simulink model "DPP_open_loop"  (R2019b)
settings: Solver=VariableStepAuto  StartTime=0.0  StopTime=3  RelTol=1e-5  EnableMultiTasking=on
libraries: powerlib x19, re_lib x2, eePwmGenerator x2, simulink x1
settings Model: Creator=Rodney Tan  LastModifiedBy=lward
settings SolverCC: ConcurrentTasks=on  ZeroCrossControl=DisableAll  AlgebraicLoopSolver=LineSearch
settings DataIOCC: LimitDataPoints=on  SaveFormat=Array  ReturnWorkspaceOutputs=off
settings OptimizationCC: LifeSpan=inf
settings DebuggingCC: SFUnexpectedBacktrackingDiag=warning  SFNoUnconditionalDefaultTransitionDiag=warning  ArithmeticOperatorsInVariantConditions=warning
settings HardwareCC: ProdBitPerPointer=32  ProdBitPerSizeT=32  ProdBitPerPtrDiffT=32  ProdLargestAtomicFloat=None  ProdIntDivRoundTo=Undefined  ProdEndianess=Unspecified  ProdWordSize=32  ProdHWDeviceType=32-bit Generic
settings ModelReferenceCC: PropagateSignalLabelsOutOfModel=off
settings SFSimCC: SimUseLocalCustomCode=off  CustomCodeUndefinedFunction=UseInterfaceOnly
settings RTWCC: RTWUseLocalCustomCode=off
settings CodeAppCC: StateflowObjectComments=on
settings GRTTargetCC: TargetLangStandard=C89/C90 (ANSI)  GeneratePreprocessorConditionals=Disable all
settings ConfigComp: CovMetricSettings=dw  CovHtmlReporting=on  CovSaveCumulativeToWorkspaceVar=on  CovSaveSingleToWorkspaceVar=on  CovExternalEMLEnable=off
settings SimscapeCC: SimscapeNormalizeSystem=off

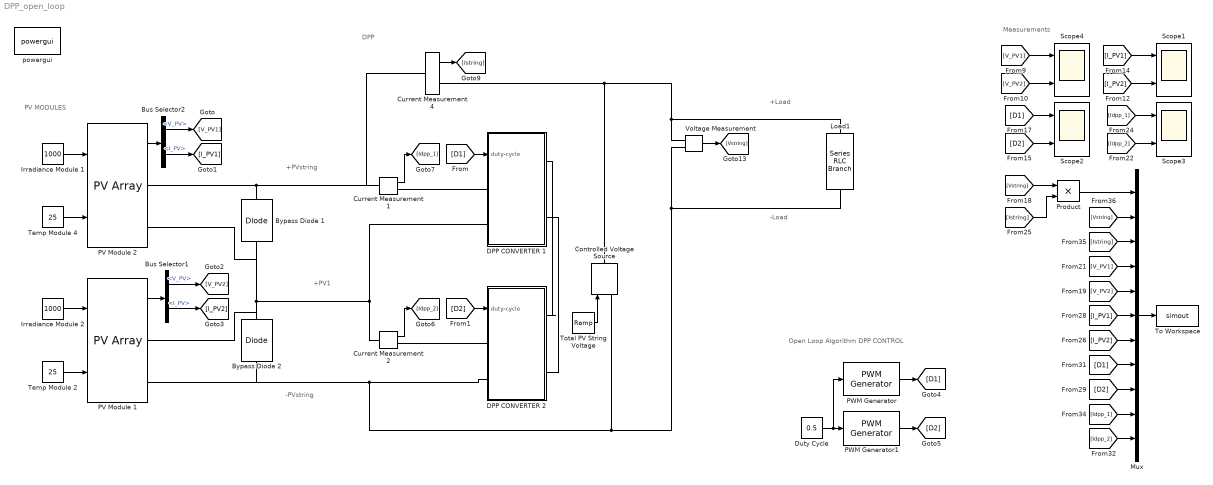
== system DPP_open_loop ==
  note: PV MODULES
  note: DPP
  note: +PV1
  note: +PVstring
  note: +Load
  note: -Load
  note: Measurements
  note: -PVstring
  note: Open Loop Algorithm
      | DPP CONTROL
  Bus Selector1 : BusSelector  OutputSignals=V_PV,I_PV
  Bus Selector2 : BusSelector  OutputSignals=V_PV,I_PV
  Bypass Diode 1 : powerlib/Power Electronics/Diode  Ron=0  Lon=0  Vf=0.8  IC=0  UseSnubber=off  Rs=0  Cs=0  Measurements=off
      settings: SourceProductName=Simscape Electrical
  Bypass Diode 2 : powerlib/Power Electronics/Diode  Ron=0  Lon=0  Vf=0.8  IC=0  UseSnubber=off  Rs=0  Cs=0  Measurements=off
      settings: SourceProductName=Simscape Electrical
  Controlled Voltage Source : powerlib/Electrical Sources/Controlled Voltage Source  Initialize=on  Source_Type=DC  Amplitude=0  Phase=0  Frequency=0  Measurements=None
      settings: SourceProductName=Simscape Electrical
  Current Measurement1 : powerlib/Measurements/Current Measurement  PhasorSimulation=off  OutputType=Complex  PSBequivalent=0
      settings: SourceProductName=Simscape Electrical
  Current Measurement2 : powerlib/Measurements/Current Measurement  PhasorSimulation=off  OutputType=Complex  PSBequivalent=0
      settings: SourceProductName=Simscape Electrical
  Current Measurement4 : powerlib/Measurements/Current Measurement  PhasorSimulation=off  OutputType=Complex  PSBequivalent=0
      settings: SourceProductName=Simscape Electrical
  DPP CONVERTER 1 : Subsystem
  DPP CONVERTER 2 : Subsystem
  Duty Cycle : Constant  Value=0.5
  Irradiance Module 1 : Constant  Value=1000
  Irradiance Module 2 : Constant  Value=1000
  Load1 : powerlib/Elements/Series RLC Branch  LConnTagsString=__new0  RConnTagsString=__new0  BranchType=R  Resistance=40  Inductance=1e-3  SetiL0=off  InitialCurrent=0  Capacitance=100e-6  Setx0=off  InitialVoltage=0  Measurements=None
      settings: SourceProductName=Simscape Electrical
  Mux : Mux  Inputs=11
  PV Module 1 : re_lib/Solar/PV Array  Npar=1  Nser=1  PlotType=array @ 1000 W/m2 & specified temperatures  S_vec="[ 1000  500  100 ]"  Temp_C_vec="[ 45 25  ]"  ModuleName=Renogy RNG-175D  PlotWhenSelected=off  Pm=175.062  Ncell=72  Voc=44.2  Isc=5.25  Vm=35.8  Im=4.89  beta_Voc_pc=-0.386  alpha_Isc_pc=0.0436  beta_Voc=-0.17061  alpha_Isc=0.002289  IL=5.2606  I0=4.127e-10  nI=1.0278  Rsh=408.404  Rs=0.58188  BAL=off  Tc=1e-6  Tfilter=5e-5
      settings: SourceProductName=Simscape Electrical
  PV Module 2 : re_lib/Solar/PV Array  Npar=1  Nser=1  PlotType=array @ 1000 W/m2 & specified temperatures  S_vec="[ 1000  500  100 ]"  Temp_C_vec="[ 45 25  ]"  ModuleName=Renogy RNG-175D  PlotWhenSelected=off  Pm=175.062  Ncell=72  Voc=44.2  Isc=5.25  Vm=35.8  Im=4.89  beta_Voc_pc=-0.386  alpha_Isc_pc=0.0436  beta_Voc=-0.17061  alpha_Isc=0.002289  IL=5.2606  I0=4.127e-10  nI=1.0278  Rsh=408.404  Rs=0.58188  BAL=off  Tc=1e-6  Tfilter=5e-5
      settings: SourceProductName=Simscape Electrical
  PWM Generator : eePwmGenerator/PWM Generator  CarrCount=Up  Tper=0.0001  Ts=1e-5
      settings: SourceProductName=Simscape Electrical
  PWM Generator1 : eePwmGenerator/PWM Generator  CarrCount=Up  Tper=0.0001  Ts=1e-5
      settings: SourceProductName=Simscape Electrical
  Product : Product
  Scope{1..4} (4 alike) : Scope  NumInputPorts=2
  Temp Module 2 : Constant  Value=25
  Temp Module 4 : Constant  Value=25
  To Workspace : ToWorkspace  VariableName=simout  SampleTime=-1
  Total PV String Voltage : simulink/Sources/Ramp  slope=50  start=0  InitialOutput=0
  Voltage Measurement : powerlib/Measurements/Voltage Measurement  PhasorSimulation=off  OutputType=Complex  PSBequivalent=0
      settings: SourceProductName=Simscape Electrical
  powergui : powerlib/powergui  Priority=1  SimulationMode=Continuous  SampleTime=1e-6  frequency=60  Iterations=50  frequencyindice=0  Pbase=100e6  ErrMax=1e-4  UnitsV=kV  UnitsW=MW  buscounter=0  FunctionMessages=off  echomessages=off  EnableUseOfTLC=off  CurrentSourceSwitches=off  DisableSnubberDevices=off  DisableRonSwitches=off  DisableVfSwitches=off  DisplayEquations=off  AutomaticDiscreteSolvers=off  SolverType=Tustin/Backward Euler (TBE)  Interpol=off  ExternalGateDelay=off  methode=off  Ts=100  x0status=blocks  SPID=off  SwTol=0  HookPort=off  NonlinearTolerance=1e-4  nMaxIteration=100  ContinueOnMaxIteration=off  RestoreLinks=warning  ResistiveCurrentMeasurement=off  Frange=[0:2:500]  Ylog=off  Xlog=on  ShowGrid=off  save=off  variable=ZData  structure=0  ZoomFFT=off  StartTime=0.0  cycles=1  DisplayStyle=1  fundamental=60  FreqAxis=off  MaxFrequency=1000  frequencyindicesteady=1  RmsSteady=1  display=off
      settings: SourceProductName=Simscape Electrical
  wires:
  Mux/1 -> To Workspace/1
  Temp Module 4/1 -> PV Module 2/2
  Irradiance Module 1/1 -> PV Module 2/1
  Temp Module 2/1 -> PV Module 1/2
  PV Module 1/1 -> Bus Selector1/1
  PV Module 2/1 -> Bus Selector2/1
  Bus Selector2/1 -> [V_PV1]  "<V_PV>"
  Bus Selector2/2 -> [I_PV1]  "<I_PV>"
  Bus Selector1/1 -> [V_PV2]  "<V_PV>"
  Bus Selector1/2 -> [I_PV2]  "<I_PV>"
  Current Measurement2/1 -> [Idpp_2]
  Current Measurement1/1 -> [Idpp_1]
  Current Measurement4/1 -> [Istring]
  [D1] -> DPP CONVERTER 1/1(duty-cycle)
  [D2] -> DPP CONVERTER 2/1(duty-cycle)
  [V_PV1] -> Scope4/1
  [V_PV2] -> Scope4/2
  [I_PV2] -> Scope1/2
  [I_PV1] -> Scope1/1
  [D2] -> Scope2/2
  [D1] -> Scope2/1
  Voltage Measurement/1 -> [Vstring]
  [Vstring] -> Product/1
  [Idpp_2] -> Scope3/2
  [Idpp_1] -> Scope3/1
  [Istring] -> Product/2
  [Idpp_2] -> Mux/11
  [Idpp_1] -> Mux/10
  Total PV String Voltage/1 -> Controlled Voltage Source/1
  Irradiance Module 2/1 -> PV Module 1/1
  [Vstring] -> Mux/2
  [Istring] -> Mux/3
  [V_PV1] -> Mux/4
  [V_PV2] -> Mux/5
  [I_PV2] -> Mux/7
  [I_PV1] -> Mux/6
  [D2] -> Mux/9
  [D1] -> Mux/8
  Product/1 -> Mux/1
  PWM Generator1/1 -> [D2]
  Duty Cycle/1 -> PWM Generator/1, PWM Generator1/1
  PWM Generator/1 -> [D1]
  connections:
  Voltage Measurement/LConn2 -- Load1/RConn1 -- Controlled Voltage Source/LConn1 -- Bypass Diode 2/LConn1 -- PV Module 1/RConn2 -- DPP CONVERTER 2/LConn2
  Current Measurement4/LConn1 -- Current Measurement1/LConn1 -- Bypass Diode 1/RConn1 -- PV Module 2/RConn1
  Current Measurement1/RConn1 -- DPP CONVERTER 1/LConn1
  DPP CONVERTER 2/LConn1 -- Current Measurement2/RConn1
  DPP CONVERTER 2/RConn2 -- DPP CONVERTER 1/RConn2
  DPP CONVERTER 2/RConn1 -- DPP CONVERTER 1/RConn1
  Voltage Measurement/LConn1 -- Load1/LConn1 -- Controlled Voltage Source/RConn1 -- Current Measurement4/RConn1
  Current Measurement2/LConn1 -- PV Module 2/RConn2 -- Bypass Diode 1/LConn1 -- PV Module 1/RConn1 -- Bypass Diode 2/RConn1 -- DPP CONVERTER 1/LConn2

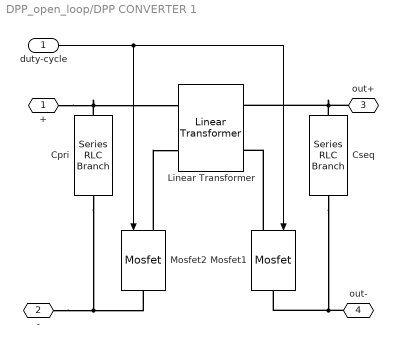
== system DPP_open_loop/DPP CONVERTER 1 ==
  duty-cycle : Inport
  Cpri : powerlib/Elements/Series RLC Branch  LConnTagsString=__new0  RConnTagsString=__new0  BranchType=RC  Resistance=100e-3  Inductance=1e-3  SetiL0=off  InitialCurrent=0  Capacitance=100e-6  Setx0=off  InitialVoltage=0  Measurements=None
      settings: SourceProductName=Simscape Electrical
  Cseq : powerlib/Elements/Series RLC Branch  LConnTagsString=__new0  RConnTagsString=__new0  BranchType=C  Resistance=1  Inductance=1e-3  SetiL0=off  InitialCurrent=0  Capacitance=100e-6  Setx0=off  InitialVoltage=0  Measurements=None
      settings: SourceProductName=Simscape Electrical
  Linear Transformer : powerlib/Elements/Linear Transformer  UNITS=SI  NominalPower=[0 0]  winding1=[1 0 0]  winding2=[1 0 0]  ThreeWindings=off  winding3=[3.15e+05 1.5753e+09 532.04]  RmLm=[inf inf]  Measurements=None  DataType=on
      settings: SourceProductName=Simscape Electrical
  Mosfet1 : powerlib/Power Electronics/Mosfet  Ron=0.1  Lon=0  Rd=0.01  Vfd=0  IC=0  Rs=1e5  Cs=inf  Measurements=off
      settings: SourceProductName=Simscape Electrical
  Mosfet2 : powerlib/Power Electronics/Mosfet  Ron=0.1  Lon=0  Rd=0.01  Vfd=0  IC=0  Rs=1e5  Cs=inf  Measurements=off
      settings: SourceProductName=Simscape Electrical
  + : PMIOPort  Side=Left
  - : PMIOPort  Port=2  Side=Left
  out+ : PMIOPort  Port=3  Side=Right
  out- : PMIOPort  Port=4  Side=Right
  wires:
  duty-cycle/1 -> Mosfet1/1, Mosfet2/1
  connections:
  Mosfet1/LConn1 -- Linear Transformer/RConn2
  Mosfet2/LConn1 -- Linear Transformer/LConn2
  -/RConn1 -- Cpri/RConn1 -- Mosfet2/RConn1
  out-/RConn1 -- Cseq/RConn1 -- Mosfet1/RConn1
  out+/RConn1 -- Cseq/LConn1 -- Linear Transformer/RConn1
  +/RConn1 -- Cpri/LConn1 -- Linear Transformer/LConn1

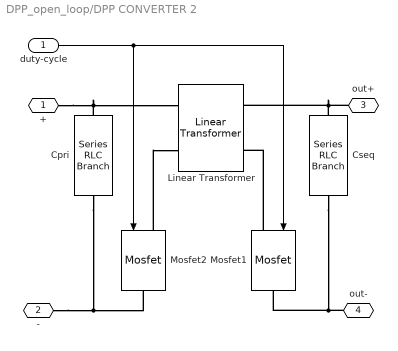
== system DPP_open_loop/DPP CONVERTER 2 ==
  duty-cycle : Inport
  Cpri : powerlib/Elements/Series RLC Branch  LConnTagsString=__new0  RConnTagsString=__new0  BranchType=RC  Resistance=100e-3  Inductance=1e-3  SetiL0=off  InitialCurrent=0  Capacitance=100e-6  Setx0=off  InitialVoltage=0  Measurements=None
      settings: SourceProductName=Simscape Electrical
  Cseq : powerlib/Elements/Series RLC Branch  LConnTagsString=__new0  RConnTagsString=__new0  BranchType=C  Resistance=1  Inductance=1e-3  SetiL0=off  InitialCurrent=0  Capacitance=100e-6  Setx0=off  InitialVoltage=0  Measurements=None
      settings: SourceProductName=Simscape Electrical
  Linear Transformer : powerlib/Elements/Linear Transformer  UNITS=SI  NominalPower=[0 0]  winding1=[1 0 0]  winding2=[1 0 0]  ThreeWindings=off  winding3=[3.15e+05 1.5753e+09 532.04]  RmLm=[inf inf]  Measurements=None  DataType=on
      settings: SourceProductName=Simscape Electrical
  Mosfet1 : powerlib/Power Electronics/Mosfet  Ron=0.1  Lon=0  Rd=0.01  Vfd=0  IC=0  Rs=1e5  Cs=inf  Measurements=off
      settings: SourceProductName=Simscape Electrical
  Mosfet2 : powerlib/Power Electronics/Mosfet  Ron=0.1  Lon=0  Rd=0.01  Vfd=0  IC=0  Rs=1e5  Cs=inf  Measurements=off
      settings: SourceProductName=Simscape Electrical
  + : PMIOPort  Side=Left
  - : PMIOPort  Port=2  Side=Left
  out+ : PMIOPort  Port=3  Side=Right
  out- : PMIOPort  Port=4  Side=Right
  wires:
  duty-cycle/1 -> Mosfet1/1, Mosfet2/1
  connections:
  Mosfet1/LConn1 -- Linear Transformer/RConn2
  Mosfet2/LConn1 -- Linear Transformer/LConn2
  -/RConn1 -- Cpri/RConn1 -- Mosfet2/RConn1
  out-/RConn1 -- Cseq/RConn1 -- Mosfet1/RConn1
  out+/RConn1 -- Cseq/LConn1 -- Linear Transformer/RConn1
  +/RConn1 -- Cpri/LConn1 -- Linear Transformer/LConn1
